simulink model "sogi_dual_output_filter_fe_validation"  (R2026a)
settings: Solver=FixedStepDiscrete  StopTime=1  FixedStep=5e-5
settings Model: DataDictionary=sogi_state_space_parameters.sldd  EnableAccessToBaseWorkspace=off  Creator=ASUS  LastModifiedBy=ASUS

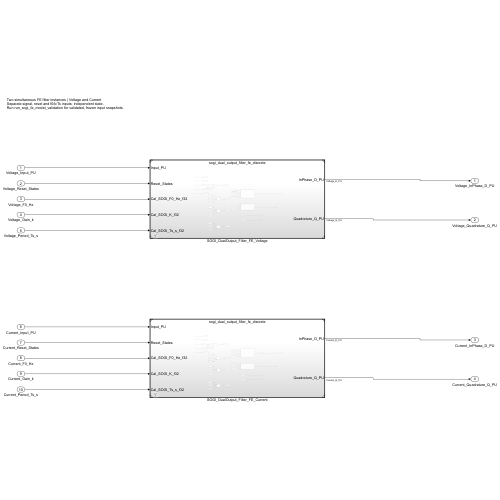
[thumbnail: Simulink's stored preview of the top-level diagram]
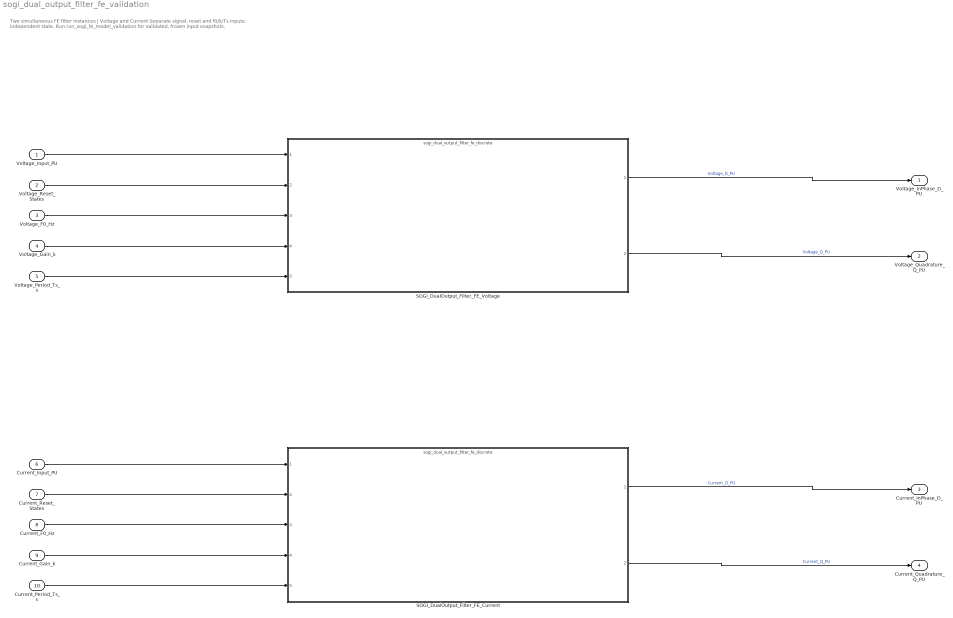
== system sogi_dual_output_filter_fe_validation ==
  note: Two simultaneous FE filter instances | Voltage and Current
      | Separate signal, reset and f0/k/Ts inputs; independent state.
      | Run run_sogi_fe_model_validation for validated, frozen input snapshots.
  Voltage_Input_PU : Inport  OutDataTypeStr=single  PortDimensions=1  Interpolate=off
  Voltage_Reset_States : Inport  Port=2  OutDataTypeStr=uint8  PortDimensions=1  Interpolate=off
  Voltage_F0_Hz : Inport  Port=3  OutDataTypeStr=single  PortDimensions=1  Interpolate=off
  Voltage_Gain_k : Inport  Port=4  OutDataTypeStr=single  PortDimensions=1  Interpolate=off
  Voltage_Period_Ts_s : Inport  Port=5  OutDataTypeStr=single  PortDimensions=1  Interpolate=off
  Current_Input_PU : Inport  Port=6  OutDataTypeStr=single  PortDimensions=1  Interpolate=off
  Current_Reset_States : Inport  Port=7  OutDataTypeStr=uint8  PortDimensions=1  Interpolate=off
  Current_F0_Hz : Inport  Port=8  OutDataTypeStr=single  PortDimensions=1  Interpolate=off
  Current_Gain_k : Inport  Port=9  OutDataTypeStr=single  PortDimensions=1  Interpolate=off
  Current_Period_Ts_s : Inport  Port=10  OutDataTypeStr=single  PortDimensions=1  Interpolate=off
  SOGI_DualOutput_Filter_FE_Current : ModelReference  ModelNameDialog=sogi_dual_output_filter_fe_discrete  SimulationMode=Normal  ModelReferenceVersion=1.1
  SOGI_DualOutput_Filter_FE_Voltage : ModelReference  ModelNameDialog=sogi_dual_output_filter_fe_discrete  SimulationMode=Normal  ModelReferenceVersion=1.1
  Voltage_InPhase_D_PU : Outport  OutDataTypeStr=single  PortDimensions=1
  Voltage_Quadrature_Q_PU : Outport  Port=2  OutDataTypeStr=single  PortDimensions=1
  Current_InPhase_D_PU : Outport  Port=3  OutDataTypeStr=single  PortDimensions=1
  Current_Quadrature_Q_PU : Outport  Port=4  OutDataTypeStr=single  PortDimensions=1
  wires:
  SOGI_DualOutput_Filter_FE_Current/2 -> Current_Quadrature_Q_PU/1  "Current_Q_PU"
  SOGI_DualOutput_Filter_FE_Current/1 -> Current_InPhase_D_PU/1  "Current_D_PU"
  Current_Period_Ts_s/1 -> SOGI_DualOutput_Filter_FE_Current/5
  Current_Gain_k/1 -> SOGI_DualOutput_Filter_FE_Current/4
  Current_F0_Hz/1 -> SOGI_DualOutput_Filter_FE_Current/3
  Current_Reset_States/1 -> SOGI_DualOutput_Filter_FE_Current/2
  Current_Input_PU/1 -> SOGI_DualOutput_Filter_FE_Current/1
  SOGI_DualOutput_Filter_FE_Voltage/2 -> Voltage_Quadrature_Q_PU/1  "Voltage_Q_PU"
  SOGI_DualOutput_Filter_FE_Voltage/1 -> Voltage_InPhase_D_PU/1  "Voltage_D_PU"
  Voltage_Period_Ts_s/1 -> SOGI_DualOutput_Filter_FE_Voltage/5
  Voltage_Gain_k/1 -> SOGI_DualOutput_Filter_FE_Voltage/4
  Voltage_F0_Hz/1 -> SOGI_DualOutput_Filter_FE_Voltage/3
  Voltage_Reset_States/1 -> SOGI_DualOutput_Filter_FE_Voltage/2
  Voltage_Input_PU/1 -> SOGI_DualOutput_Filter_FE_Voltage/1
